simulink model "MotorControllerwithStateSpaceSimulink"  (R2020a)
settings: Solver=VariableStepAuto  StartTime=0.0  StopTime=10.0  RelTol=1e-3
settings Model: Creator=Oguzhan  LastModifiedBy=oguzhan
settings DataIOCC: ReturnWorkspaceOutputs=off
settings DebuggingCC: ArithmeticOperatorsInVariantConditions=warning
settings SFSimCC: SimUseLocalCustomCode=off  CustomCodeUndefinedFunction=UseInterfaceOnly
settings RTWCC: RTWUseLocalCustomCode=off

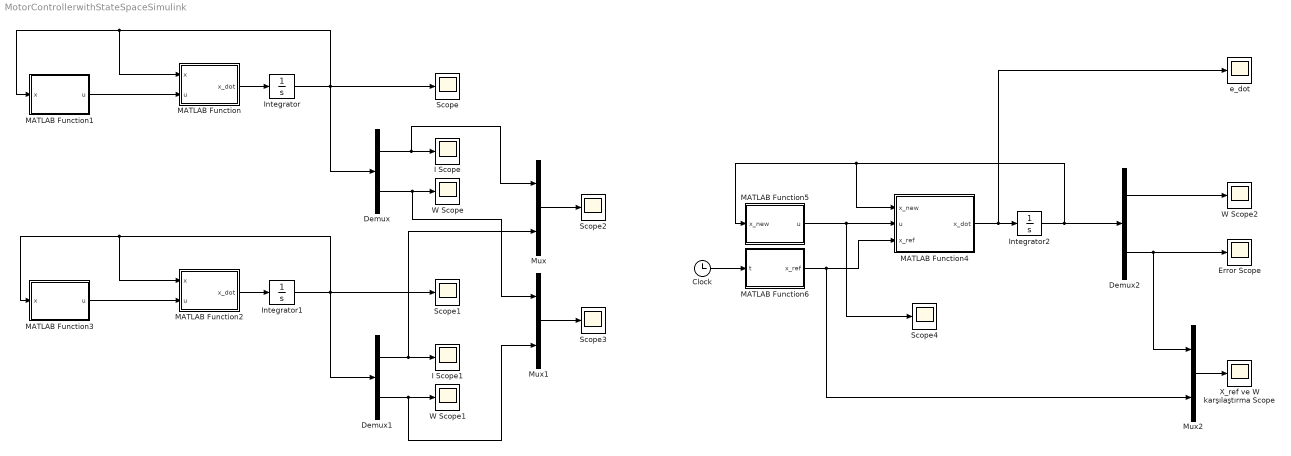
== system MotorControllerwithStateSpaceSimulink ==
  Clock : Clock
  Demux : Demux  Outputs=2
  Demux1 : Demux  Outputs=2
  Demux2 : Demux  Outputs=2
  Error Scope : Scope
  I Scope : Scope
  I Scope1 : Scope
  Integrator : Integrator  InitialCondition=[100,20]
  Integrator1 : Integrator  InitialCondition=[100,20]
  Integrator2 : Integrator  InitialCondition=[0,50,0]
  MATLAB Function : MATLAB Function  TreatAsAtomicUnit=on
  MATLAB Function1 : MATLAB Function  TreatAsAtomicUnit=on
  MATLAB Function2 : MATLAB Function  TreatAsAtomicUnit=on
  MATLAB Function3 : MATLAB Function  TreatAsAtomicUnit=on
  MATLAB Function4 : MATLAB Function  TreatAsAtomicUnit=on
  MATLAB Function5 : MATLAB Function  TreatAsAtomicUnit=on
  MATLAB Function6 : MATLAB Function  TreatAsAtomicUnit=on
  Mux : Mux  Inputs=2
  Mux1 : Mux  Inputs=2
  Mux2 : Mux  Inputs=2
  Scope{,1..4} (5 alike) : Scope
  W Scope : Scope
  W Scope1 : Scope
  W Scope2 : Scope
  X_ref ve W karşılaştırma Scope : Scope
  e_dot : Scope
  wires:
  MATLAB Function/1(x_dot) -> Integrator/1
  Integrator/1 -> Scope/1, MATLAB Function1/1(x), MATLAB Function/1(x), Demux/1
  MATLAB Function1/1(u) -> MATLAB Function/2(u)
  Demux/1 -> Mux/1, I Scope/1
  Demux/2 -> Mux1/1, W Scope/1
  Demux1/1 -> Mux/2, I Scope1/1
  MATLAB Function3/1(u) -> MATLAB Function2/2(u)
  Integrator1/1 -> Scope1/1, MATLAB Function3/1(x), MATLAB Function2/1(x), Demux1/1
  MATLAB Function2/1(x_dot) -> Integrator1/1
  Demux1/2 -> W Scope1/1, Mux1/2
  Mux/1 -> Scope2/1
  Mux1/1 -> Scope3/1
  MATLAB Function6/1(x_ref) -> Mux2/2, MATLAB Function4/3(x_ref)
  MATLAB Function4/1(x_dot) -> e_dot/1, Integrator2/1
  Mux2/1 -> X_ref ve W karşılaştırma Scope/1
  Demux2/2 -> Error Scope/1, Mux2/1
  Demux2/1 -> W Scope2/1
  MATLAB Function5/1(u) -> Scope4/1, MATLAB Function4/2(u)
  Clock/1 -> MATLAB Function6/1(t)
  Integrator2/1 -> Demux2/1, MATLAB Function5/1(x_new), MATLAB Function4/1(x_new)

== matlab function MotorControllerwithStateSpaceSimulink/MATLAB Function ==
  data: x input; u input; x_dot output
function x_dot = fcn(x,u)

J = 0.09;
K = 85*10^-3;
R = 0.55;
b = 0.05;
L = 25*10^-3;

a11 = -R/L;
a12 = -K/L;
a21 = K/J;
a22 = -b/J;

b11 = 1/L;
b21 = 0;

A = [a11,a12;
     a21,a22];
 
B = [b11;
     b21];
 
x_dot = A*x + B*u;

end

== matlab function MotorControllerwithStateSpaceSimulink/MATLAB Function2 ==
  data: x input; u input; x_dot output
function x_dot = fcn(x,u)

J = 0.09;
K = 85*10^-3;
R = 0.55;
b = 0.05;
L = 25*10^-3;

a11 = -R/L;
a12 = -K/L;
a21 = K/J;
a22 = -b/J;

b11 = 1/L;
b21 = 0;

A = [a11,a12;
     a21,a22];
 
B = [b11;
     b21];
 
x_dot = A*x ;

end

== matlab function MotorControllerwithStateSpaceSimulink/MATLAB Function3 ==
  data: x input; u output
function u = fcn(x)

% U = -K.x olduğu için x'e yani statelere bağlıdır. K ise sadece bir değişkendir.

K = [-0.3389    0.3202]; %-4 ve -5 ' a göre K parametresinin sonuçları.
u = -K*x; % Bu sisteme her giriş verdiğimde bu response ı verir.

end

== matlab function MotorControllerwithStateSpaceSimulink/MATLAB Function4 ==
  data: x_new input; u input; x_dot output; x_ref input
function x_dot = fcn(x_new,u,x_ref)

 J = 0.09;
 K = 85*10^-3;
 R = 0.55;
 b = 0.05;
 L = 25*10^-3;

 a11 = -R/L;
 a12 = -K/L;
 a21 = K/J;
 a22 = -b/J;

 b11 = 1/L;
 b21 = 0;

 A = [a11,a12;
      a21,a22];
 
 B = [b11;
      b21];

 A_new = [A,zeros(2,1);
          0, 1, 0];
      
 B_new = [B; 
          0];
 
 E_ref =  [0; 
           0;
           -1];   

x_dot = A_new*x_new + B_new*u + E_ref*x_ref;

end

== matlab function MotorControllerwithStateSpaceSimulink/MATLAB Function5 ==
  data: x_new input; u output
function u = fcn(x_new)

%K = [0.5611   16.4673   79.4118]; %20, 15, 10 Daha yavaş bir sistem
%K = 10^3*[0.0043    0.3319    7.2265];  %-70,-65,-60 hızlı bir sistem
K = 10^4*[0.0011    0.1714    7.9412] %Çok çok daha hızlı

u = -K*x_new;

end

== matlab function MotorControllerwithStateSpaceSimulink/MATLAB Function6 ==
  data: t input; x_ref output
function x_ref = fcn(t)

bias = 50;
A = 5;%+-5 rpm
f = 1;% 1 Hz

x_ref = bias + A*sin(2*pi*f*t);

end

== matlab function MotorControllerwithStateSpaceSimulink/MATLAB Function1 ==
  data: x input; u output
function u = fcn(x)

% U = -K.x olduğu için x'e yani statelere bağlıdır. K ise sadece bir değişkendir.

K = [1.1861   30.6585]; %-30 ve -40 ' a göre K parametresinin sonuçları.
u = -K*x; % Bu sisteme her giriş verdiğimde bu response ı verir.

end
